simulink model "first"  (Simulink 7.2)
settings: Solver=ode15s  StartTime=0.0  StopTime=2  RelTol=1e-3
libraries: powerlib x22, powerlib_extras x6
settings Model: Creator=User  LastModifiedBy=hamed
settings DataIOCC: SaveFormat=StructureWithTime

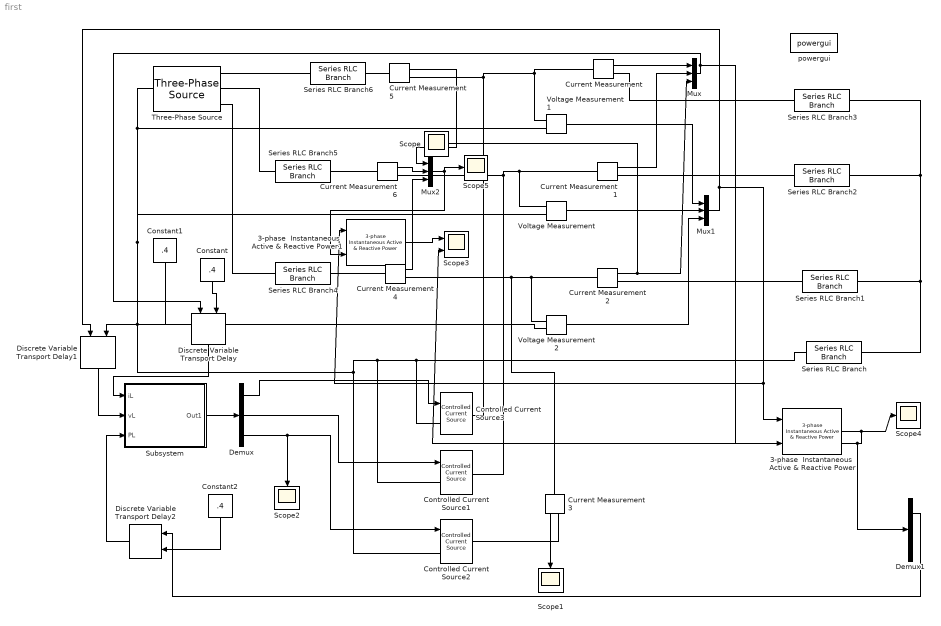
== system first ==
  3-phase  Instantaneous  Active & Reactive Power : powerlib_extras/Measurements/3-phase  Instantaneous  Active & Reactive Power  DialogController=POWERSYS.PowerSysDialog  SystemSampleTime=-1
  3-phase  Instantaneous  Active & Reactive Power1 : powerlib_extras/Measurements/3-phase  Instantaneous  Active & Reactive Power  DialogController=POWERSYS.PowerSysDialog  SystemSampleTime=-1
  Constant : Constant  Orientation=down  Value=.4  OutDataType=sfix(16)  OutScaling=2^0
  Constant1 : Constant  Orientation=down  Value=.4  OutDataType=sfix(16)  OutScaling=2^0
  Constant2 : Constant  Orientation=down  Value=.4  OutDataType=sfix(16)  OutScaling=2^0
  Controlled Current Source1 : powerlib/Electrical Sources/Controlled Current Source  DialogController=POWERSYS.PowerSysDialog  SystemSampleTime=-1  Initialize=on  Source_Type=AC  Amplitude=0  Phase=0  Frequency=0  Measurements=None
  Controlled Current Source2 : powerlib/Electrical Sources/Controlled Current Source  DialogController=POWERSYS.PowerSysDialog  SystemSampleTime=-1  Initialize=on  Source_Type=AC  Amplitude=0  Phase=0  Frequency=0  Measurements=None
  Controlled Current Source3 : powerlib/Electrical Sources/Controlled Current Source  DialogController=POWERSYS.PowerSysDialog  SystemSampleTime=-1  Initialize=on  Source_Type=AC  Amplitude=0  Phase=0  Frequency=0  Measurements=None
  Current Measurement{,1..2,4..6} (6 alike) : powerlib/Measurements/Current Measurement  DialogController=POWERSYS.PowerSysDialog  SystemSampleTime=-1  PhasorSimulation=off  OutputType=Complex  PSBequivalent=0
  Current Measurement3 : powerlib/Measurements/Current Measurement  Orientation=down  DialogController=POWERSYS.PowerSysDialog  SystemSampleTime=-1  PhasorSimulation=off  OutputType=Complex  PSBequivalent=0
  Demux : Demux  Outputs=3
  Demux1 : Demux  Outputs=2
  Discrete Variable Transport Delay : powerlib_extras/Discrete  Control Blocks/Discrete Variable Transport Delay  Orientation=down  DialogController=POWERSYS.PowerSysDialog  SystemSampleTime=-1  MaxDelay=1/40  InitialValue=0  Ts=50e-6
  Discrete Variable Transport Delay1 : powerlib_extras/Discrete  Control Blocks/Discrete Variable Transport Delay  Orientation=down  DialogController=POWERSYS.PowerSysDialog  SystemSampleTime=-1  MaxDelay=1/40  InitialValue=0  Ts=50e-6
  Discrete Variable Transport Delay2 : powerlib_extras/Discrete  Control Blocks/Discrete Variable Transport Delay  Orientation=left  DialogController=POWERSYS.PowerSysDialog  SystemSampleTime=-1  MaxDelay=1/40  InitialValue=0  Ts=50e-6
  Mux : Mux  Inputs=3
  Mux1 : Mux  Inputs=3
  Mux2 : Mux  Inputs=3
  Scope{,1..2,4..5} (5 alike) : Scope
      Scope settings: TimeRange=2  YMin=-125  YMax=200  SaveName=ScopeData2
      Scope1 settings: Orientation=down  TimeRange=0.06  YMin=-1e-010  YMax=1e-010  SaveName=ScopeData3
      Scope2 settings: Orientation=down  TimeRange=0.5  YMin=-100  YMax=200  SaveName=ScopeData4
      Scope4 settings: TimeRange=2  YMin=-25000  YMax=200000  SaveName=ScopeData8
      Scope5 settings: TimeRange=0.2  YMin=-125  YMax=125  SaveName=ScopeData5
  Scope3 : Scope  NumInputPorts=2
      settings: TimeRange=2  YMin=-10000~-25000  YMax=60000~125000  SaveName=ScopeData6
  Series RLC Branch{,4..6} (4 alike) : powerlib/Elements/Series RLC Branch  DialogController=POWERSYS.PowerSysDialog  PhysicalDomain=powersysdomain  SubClassName=unknown  LeftPortType=p1  RightPortType=p1  LConnTagsString=__new0  RConnTagsString=__new0  BranchType=R  Resistance=1  Inductance=1.0  SetiL0=off  InitialCurrent=0  Capacitance=1.0  Setx0=off  InitialVoltage=0  Measurements=None
  Series RLC Branch1 : powerlib/Elements/Series RLC Branch  DialogController=POWERSYS.PowerSysDialog  PhysicalDomain=powersysdomain  SubClassName=unknown  LeftPortType=p1  RightPortType=p1  LConnTagsString=__new0  RConnTagsString=__new0  BranchType=R  Resistance=2  Inductance=1.0  SetiL0=off  InitialCurrent=0  Capacitance=1.0  Setx0=off  InitialVoltage=0  Measurements=None
  Series RLC Branch2 : powerlib/Elements/Series RLC Branch  DialogController=POWERSYS.PowerSysDialog  PhysicalDomain=powersysdomain  SubClassName=unknown  LeftPortType=p1  RightPortType=p1  LConnTagsString=__new0  RConnTagsString=__new0  BranchType=R  Resistance=2  Inductance=1.0  SetiL0=off  InitialCurrent=0  Capacitance=1.0  Setx0=off  InitialVoltage=0  Measurements=None
  Series RLC Branch3 : powerlib/Elements/Series RLC Branch  DialogController=POWERSYS.PowerSysDialog  PhysicalDomain=powersysdomain  SubClassName=unknown  LeftPortType=p1  RightPortType=p1  LConnTagsString=__new0  RConnTagsString=__new0  BranchType=R  Resistance=2  Inductance=1.0  SetiL0=off  InitialCurrent=0  Capacitance=1.0  Setx0=off  InitialVoltage=0  Measurements=None
  Subsystem : Subsystem
  Three-Phase Source : powerlib/Electrical Sources/Three-Phase Source  DialogController=POWERSYS.PowerSysDialog  SystemSampleTime=-1  Voltage=380  PhaseAngle=0  Frequency=50  InternalConnection=Yn  SpecifyImpedance=on  Resistance=0.8929  Inductance=16.58e-3  ShortCircuitLevel=100e6  BaseVoltage=380  XRratio=7
  Voltage Measurement : powerlib/Measurements/Voltage Measurement  DialogController=POWERSYS.PowerSysDialog  SystemSampleTime=-1  PhasorSimulation=off  OutputType=Complex  PSBequivalent=0
  Voltage Measurement1 : powerlib/Measurements/Voltage Measurement  DialogController=POWERSYS.PowerSysDialog  SystemSampleTime=-1  PhasorSimulation=off  OutputType=Complex  PSBequivalent=0
  Voltage Measurement2 : powerlib/Measurements/Voltage Measurement  DialogController=POWERSYS.PowerSysDialog  SystemSampleTime=-1  PhasorSimulation=off  OutputType=Complex  PSBequivalent=0
  powergui : powerlib/powergui  SystemSampleTime=-1  SimulationMode=Continuous  SampleTime=50e-6  frequency=60  SPID=off  DisableSnubberDevices=off  DisableRonSwitches=off  DisableVfSwitches=off  SwTol=0  Interpol=off  frequencyindice=0  echomessages=off  HookPort=off  FunctionMessages=off  EnableUseOfTLC=off  x0status=blocks  RestoreLinks=warning  Frange=[0:2:500]  Ylog=off  Xlog=on  ShowGrid=off  save=off  variable=ZData  ZoomFFT=on  StartTime=0.0  cycles=1  DisplayStyle=1  fundamental=60  FreqAxis=off  MaxFrequency=1000  frequencyindicesteady=1  RmsSteady=1  display=off  Ts=0  methode=off
  wires:
  Current Measurement1/1 -> Mux/2
  Current Measurement2/1 -> Mux/3, Scope/1
  Voltage Measurement/1 -> Mux1/2
  Voltage Measurement2/1 -> Mux1/3
  Voltage Measurement1/1 -> Mux1/1
  Demux/1 -> Controlled Current Source3/1
  Demux/2 -> Controlled Current Source1/1
  Demux/3 -> Controlled Current Source2/1, Scope2/1
  Current Measurement3/1 -> Scope1/1
  Current Measurement/1 -> Mux/1
  Discrete Variable Transport Delay/1 -> Subsystem/1(iL)
  Mux/1 -> Discrete Variable Transport Delay/1, 3-phase  Instantaneous  Active & Reactive Power/2
  Constant/1 -> Discrete Variable Transport Delay/2
  Discrete Variable Transport Delay1/1 -> Subsystem/2(vL)
  Mux1/1 -> Discrete Variable Transport Delay1/1, 3-phase  Instantaneous  Active & Reactive Power/1, 3-phase  Instantaneous  Active & Reactive Power1/1
  Constant1/1 -> Discrete Variable Transport Delay1/2
  3-phase  Instantaneous  Active & Reactive Power/1 -> Scope4/1, Scope3/2, Demux1/1
  Current Measurement5/1 -> Mux2/1
  Current Measurement6/1 -> Mux2/2
  Current Measurement4/1 -> Mux2/3
  3-phase  Instantaneous  Active & Reactive Power1/1 -> Scope3/1
  Mux2/1 -> 3-phase  Instantaneous  Active & Reactive Power1/2, Scope5/1
  Subsystem/1(Out1) -> Demux/1
  Demux1/1 -> Discrete Variable Transport Delay2/1
  Discrete Variable Transport Delay2/1 -> Subsystem/3(PL)
  Constant2/1 -> Discrete Variable Transport Delay2/2
  connections:
  Controlled Current Source3/RConn1 -- Current Measurement/LConn1 -- Voltage Measurement1/LConn1 -- Current Measurement5/RConn1
  Series RLC Branch/LConn1 -- Controlled Current Source3/LConn1 -- Controlled Current Source1/LConn1 -- Voltage Measurement/LConn2 -- Three-Phase Source/LConn1 -- Voltage Measurement1/LConn2 -- Voltage Measurement2/LConn2 -- Controlled Current Source2/LConn1
  Current Measurement3/LConn1 -- Current Measurement2/LConn1 -- Voltage Measurement2/LConn1 -- Current Measurement4/RConn1
  Current Measurement1/RConn1 -- Series RLC Branch2/LConn1
  Current Measurement2/RConn1 -- Series RLC Branch1/LConn1
  Series RLC Branch3/RConn1 -- Series RLC Branch/RConn1 -- Series RLC Branch1/RConn1 -- Series RLC Branch2/RConn1
  Current Measurement/RConn1 -- Series RLC Branch3/LConn1
  Series RLC Branch6/LConn1 -- Three-Phase Source/RConn1
  Three-Phase Source/RConn2 -- Series RLC Branch5/LConn1
  Three-Phase Source/RConn3 -- Series RLC Branch4/LConn1
  Controlled Current Source2/RConn1 -- Current Measurement3/RConn1
  Current Measurement4/LConn1 -- Series RLC Branch4/RConn1
  Current Measurement5/LConn1 -- Series RLC Branch6/RConn1
  Current Measurement6/LConn1 -- Series RLC Branch5/RConn1
  Controlled Current Source1/RConn1 -- Current Measurement1/LConn1 -- Voltage Measurement/LConn1 -- Current Measurement6/RConn1

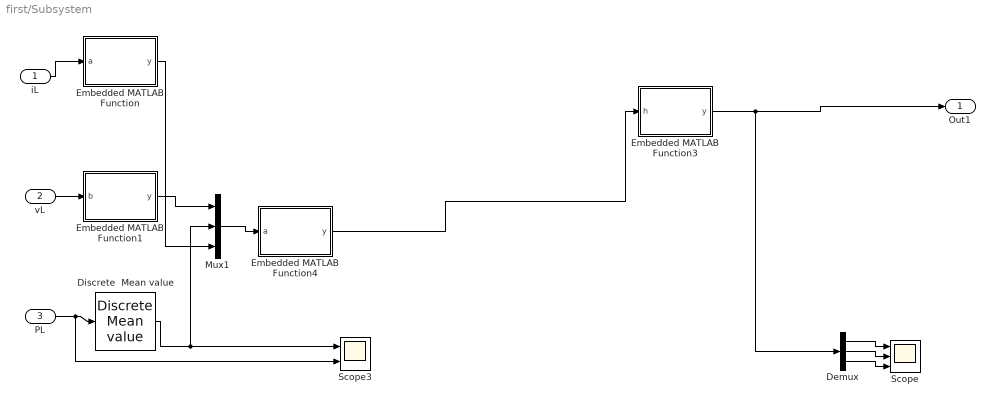
== system first/Subsystem ==
  iL : Inport  OutDataType=fixdt(1, 16)  OutScaling=2^0
  vL : Inport  Port=2  OutDataType=fixdt(1, 16)  OutScaling=2^0
  PL : Inport  Port=3  OutDataType=fixdt(1, 16)  OutScaling=2^0
  Demux : Demux  Outputs=3
  Discrete  Mean value : powerlib_extras/Discrete Measurements/Discrete  Mean value  DialogController=POWERSYS.PowerSysDialog  SystemSampleTime=-1  Freq=50  Vinit=.001  Ts=50e-6
  Embedded MATLAB Function : Stateflow chart  TreatAsAtomicUnit=on
  Embedded MATLAB Function1 : Stateflow chart  TreatAsAtomicUnit=on
  Embedded MATLAB Function3 : Stateflow chart  TreatAsAtomicUnit=on
  Embedded MATLAB Function4 : Stateflow chart  TreatAsAtomicUnit=on
  Mux1 : Mux  Inputs=3
  Scope : Scope  NumInputPorts=3
      settings: YMin=-1~-1~-1  YMax=1~1~1
  Scope3 : Scope  NumInputPorts=2
      settings: YMin=-150~-150  YMax=150~150  SaveName=ScopeData9
  Out1 : Outport  OutDataType=sfix(16)  OutScaling=2^0
  wires:
  vL/1 -> Embedded MATLAB Function1/1(b)
  Embedded MATLAB Function/1(y) -> Mux1/3
  Demux/1 -> Scope/1
  Demux/2 -> Scope/2
  Demux/3 -> Scope/3
  Embedded MATLAB Function1/1(y) -> Mux1/1
  iL/1 -> Embedded MATLAB Function/1(a)
  PL/1 -> Discrete  Mean value/1, Scope3/2
  Discrete  Mean value/1 -> Scope3/1, Mux1/2
  Mux1/1 -> Embedded MATLAB Function4/1(a)
  Embedded MATLAB Function4/1(y) -> Embedded MATLAB Function3/1(h)
  Embedded MATLAB Function3/1(y) -> Out1/1, Demux/1

== matlab function Subsystem/Embedded MATLAB Function ==
  data: a input double; y output double
function y = fcn(a)
%#eml

y =[1/sqrt(3) 1/sqrt(3) 1/sqrt(3); sqrt(2)/sqrt(3) -sqrt(2)/(2*sqrt(3)) -sqrt(2)/(2*sqrt(3)); 0 1/sqrt(2) -1/sqrt(2)]*a;

== matlab function Subsystem/Embedded MATLAB Function1 ==
  data: b input double; y output double
function y = fcn(b)
%#eml

y = [1/sqrt(3) 1/sqrt(3) 1/sqrt(3); sqrt(2)/sqrt(3) -sqrt(2)/(2*sqrt(3)) -sqrt(2)/(2*sqrt(3)); 0 1/sqrt(2) -1/sqrt(2)]*b;

== matlab function Subsystem/Embedded MATLAB Function3 ==
  data: h input double; y output double
function y = fcn(h)
%#eml

y =[1/sqrt(3) sqrt(2)/sqrt(3) 0 ;1/sqrt(3) -sqrt(2)/(2*sqrt(3)) 1/sqrt(2) ;1/sqrt(3) -sqrt(2)/(2*sqrt(3)) -1/sqrt(2)]*h;

== matlab function Subsystem/Embedded MATLAB Function4 ==
  data: a input double; y output double
function y = fcn(a)
% #eml
if (a(2)^2+a(3)^2)==0
    y=[0; 0;0];
else
y =-[0;a(2);a(3)]*(a(4)/(a(2)^2+a(3)^2))+[a(5);a(6);a(7)];
end
